simulink model "p1q67"  (R2021b)
settings: Solver=VariableStepAuto  StartTime=0.0  StopTime=100e-3  MaxStep=1e-6  RelTol=1e-3
values from neighbouring files (symbols this model uses):
  Q5 =     [part1.mat]
libraries: cstblocks x6
settings Model: Creator=najja  LastModifiedBy=bryan
settings SolverCC: AlgebraicLoopSolver=TrustRegion
settings DebuggingCC: SFMachineParentedDataDiag=warning

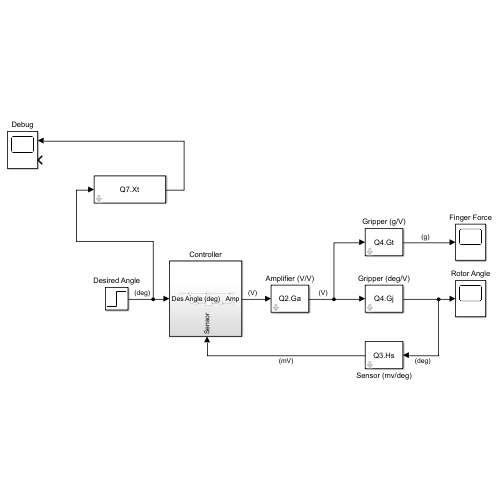
[thumbnail: Simulink's stored preview of the top-level diagram]
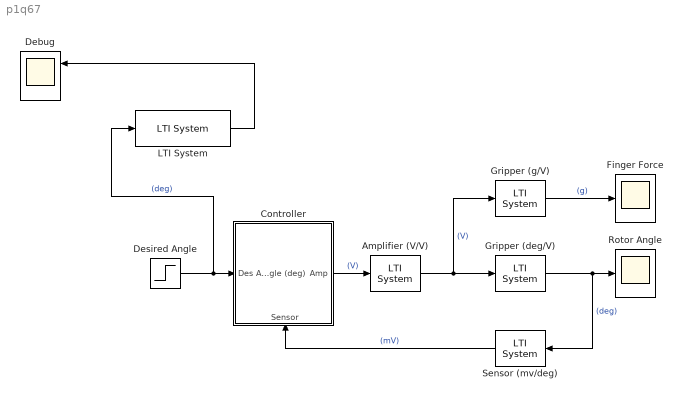
== system p1q67 ==
  Amplifier (V/V) : cstblocks/LTI System  sys=Q2.Ga  IC=[]
  Controller : Subsystem
      settings: PortSchema="{\"entries\":[{\"content\":{\"sides\":[{\"content\":{\"connectorIds\":[\"In1\"]},\"type\":\"ConnectorPlacement.EquallySpacedRectSide\",\"uuid\":\"20a6f550-8556-4a95-ba97-0f0d038d1d17\"},{\"content\":{\"connectorIds\":[\"Out1\"],\"side\":\"RIGHT\"},\"type\":\"ConnectorPlacement.EquallySpacedRectSide\",\"uuid\":\"637ee4cd-983b-493c-a336-69ccf94ca87f\"},{\"content\":{\"connectorIds\":[],\"side\":\"TOP\"},\"type\":\"ConnectorPlacement.EquallySpacedRectSide\",\"uuid\":\"29997b73-0934-4e5b-b714-2483ad9b2c52\"},{\"content\":{\"connectorIds\":[\"In2\"],\"side\":\"BOTTOM\"},\"type\":\"ConnectorPlacement.EquallySpacedRectSide\",\"uuid\":\"ddd46aa8-eb9b-4722-9811-63f8f0fb585c\"}]},\"type\":\"ConnectorPlacement.EquallySpacedConnector\",\"uuid\":\"f3289d56-3384-4f14-8545-916a0d15ea51\"}],\"packageUris\":[\"http://schema.mathworks.com/mf0/Connector/R2020b\"],\"version\":\"1.0\"}"
  Debug : Scope  NumInputPorts=2
  Desired Angle : Step  Time=0  After=120  SampleTime=0
  Finger Force : Scope
  Gripper (deg/V) : cstblocks/LTI System  sys=Q4.Gj  IC=[]
  Gripper (g/V) : cstblocks/LTI System  sys=Q4.Gt  IC=[]
  LTI System : cstblocks/LTI System  sys=Q7.Xt  IC=[]
  Rotor Angle : Scope
  Sensor (mv/deg) : cstblocks/LTI System  sys=Q3.Hs  IC=[]
  wires:
  Amplifier (V/V)/1 -> Gripper (g/V)/1, Gripper (deg/V)/1  "(V)"
  Gripper (deg/V)/1 -> Sensor (mv/deg)/1, Rotor Angle/1  "(deg)"
  Desired Angle/1 -> LTI System/1, Controller/1(Des Angle (deg))  "(deg)"
  Sensor (mv/deg)/1 -> Controller/2(Sensor)  "(mV)"
  Controller/1(Amp) -> Amplifier (V/V)/1  "(V)"
  Gripper (g/V)/1 -> Finger Force/1  "(g)"
  LTI System/1 -> Debug/1

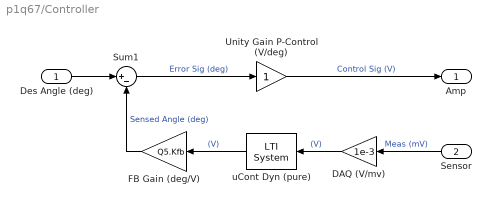
== system p1q67/Controller ==
  Des Angle (deg) : Inport
  Sensor : Inport  Port=2
  DAQ (V/mv) : Gain  Gain=1e-3
  FB Gain (deg/V) : Gain  Gain=Q5.Kfb
  Sum1 : Sum  Inputs=|+-
  Unity Gain P-Control (V/deg) : Gain
  uCont Dyn (pure) : cstblocks/LTI System  sys=Q5.Du  IC=[]
  Amp : Outport
  wires:
  FB Gain (deg/V)/1 -> Sum1/2  "Sensed Angle (deg)"
  Des Angle (deg)/1 -> Sum1/1
  Sensor/1 -> DAQ (V/mv)/1  "Meas (mV)"
  Sum1/1 -> Unity Gain P-Control (V/deg)/1  "Error Sig (deg)"
  uCont Dyn (pure)/1 -> FB Gain (deg/V)/1  "(V)"
  Unity Gain P-Control (V/deg)/1 -> Amp/1  "Control Sig (V)"
  DAQ (V/mv)/1 -> uCont Dyn (pure)/1  "(V)"
